simulink model "model"  (R2018a)
settings: Solver=VariableStepAuto  StartTime=0.0  StopTime=10.0  RelTol=1e-3
undefined symbols (not defined in the file or in its folder): magnitude
libraries: simulink x1
settings Model: Creator=maroufi  LastModifiedBy=maroufi

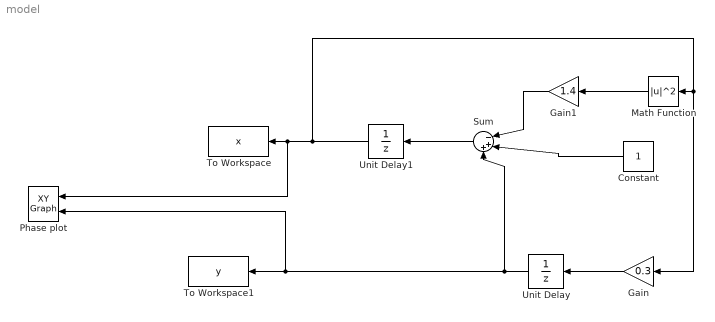
== system model ==
  Constant : Constant
  Gain : Gain  Gain=0.3
  Gain1 : Gain  Gain=1.4
  Math Function : Math  Operator=magnitude^2  SaturateOnIntegerOverflow=on
  Phase plot : simulink/Sinks/XY Graph  xmin=-1  xmax=1  ymin=-1  ymax=1  st=-1
  Sum : Sum  Inputs=|-++
  To Workspace : ToWorkspace  VariableName=x  SaveFormat=Timeseries  SampleTime=-1
  To Workspace1 : ToWorkspace  VariableName=y  SaveFormat=Timeseries  SampleTime=-1
  Unit Delay : UnitDelay  InitialCondition=1  SampleTime=-1
  Unit Delay1 : UnitDelay  InitialCondition=1  SampleTime=-1
  wires:
  Constant/1 -> Sum/2
  Gain/1 -> Unit Delay/1
  Unit Delay/1 -> Phase plot/2, To Workspace1/1, Sum/3
  Gain1/1 -> Sum/1
  Sum/1 -> Unit Delay1/1
  Unit Delay1/1 -> Gain/1, Math Function/1, Phase plot/1, To Workspace/1
  Math Function/1 -> Gain1/1
